simulink model "pert_test"  (R2021a)
settings: Solver=VariableStepAuto  StartTime=0.0  StopTime=10.0  RelTol=1e-3
libraries: spsDistributedParametersLineLib x23, spsThreePhaseSeriesRLCLoadLib x10, spsThreePhaseVIMeasurementLib x2, spsGroundLib x1, spsThreePhaseSourceLib x1, spsSeriesRLCBranchLib x1, spspowerguiLib x1
settings Model: Creator=Admin  LastModifiedBy=Admin

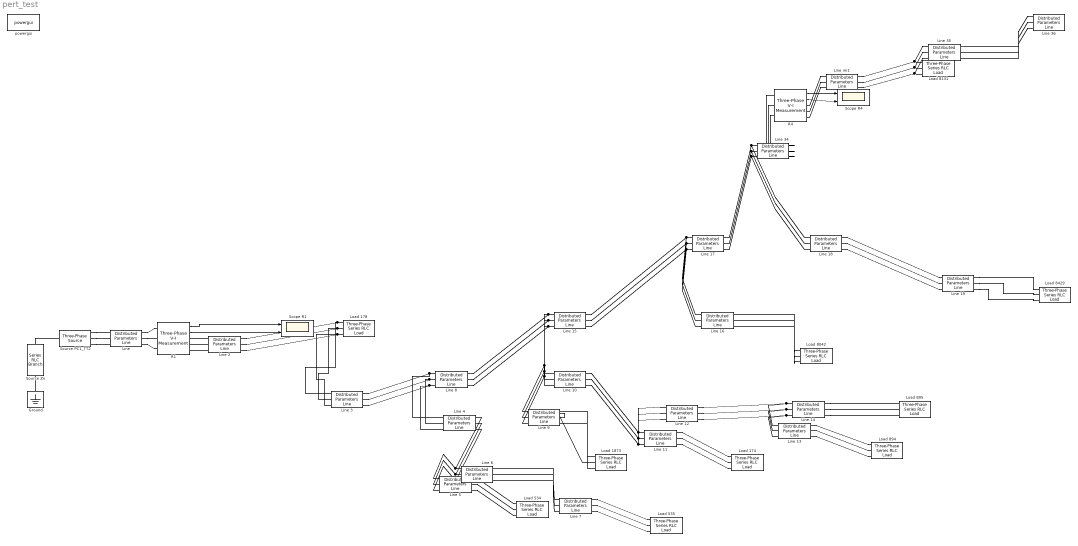
== system pert_test ==
  Ground : spsGroundLib/Ground  LConnTagsString=a
  Line : spsDistributedParametersLineLib/Distributed Parameters Line  Phases=3  Length=0.01  Frequency=50  Resistance=[0.476003738225748 0.351747138225748 0.351747138225748;0.351747138225748 0.476003738225748 0.351747138225748;0.351747138225748 0.351747138225748 0.476003738225748]  Inductance=[0.000705954362986426 0.000459934243504405 0.000459934243504405;0.000459934243504405 0.000705954362986426 0.000459934243504405;0.000459934243504405 0.000459934243504405 0.000705954362986426]  Capacitance=[5.7561313269996e-07 -1.37543883484145e-07 -1.37543912800485e-07;-1.37543883484145e-07 5.75613027339387e-07 -1.37543875208088e-07;-1.37543912800485e-07 -1.37543875208088e-07 5.75613005057695e-07]  x1=[0.0411142303390509 8948.31210962418 8947.00376137828;314.159265358979 314.159265358979 314.159265358979;0.611923927431942 -0.18676884033554 -1.75807236900485]  x2=[0.0414032445747134 8946.36312269012 8945.04836899278;314.159265358979 314.159265358979 314.159265358979;0.601696966026441 -0.186737497564286 -1.75804144074362]  x3=[0.0398944700946316 1024.91732359745 1027.78972143796;314.159265358979 314.159265358979 314.159265358979;-0.758331171111026 1.94809969608719 0.380951756978552]  x4=[0.0396805412633415 1741.95820546104 1746.36504307517;314.159265358979 314.159265358979 314.159265358979;2.35558471923768 -0.707167616201734 -2.27711571538718]  x5=2.2104317621921e-07  V1=[9.635 6853 6854;314.2 314.2 314.2;-1.242 -0.5939 -2.165]  V2=[9.699 6846 6847;314.2 314.2 314.2;-1.252 -0.5942 -2.166]  I1=[9.527 4746 4750;314.2 314.2 314.2;-2.657 2.284 0.7135]  I2=[9.488 5462 5466;314.2 314.2 314.2;0.457 -0.8227 -2.393]  nHarmo=1  Measurements=None  Decoupling=off  VsMag0=0  VrMag0=0  VsAngle0=0  VrAngle0=0  IsMag0=0  IrMag0=0  IsAngle0=0  IrAngle0=0
      settings: SourceProductBaseCode=PS
  Line 10 : spsDistributedParametersLineLib/Distributed Parameters Line  Phases=3  Length=0.16001  Frequency=50  Resistance=[0.646656091154803 0.0486237908083191 0.0486712220507153;0.0486237908083191 0.646561225344642 0.0486237934466192;0.0486712220507153 0.0486237934466192 0.646656091154803]  Inductance=[0.00282448912315926 0.00133270803418135 0.00132951476746136;0.00133270803418135 0.00282479813276775 0.00133799988507366;0.00132951476746136 0.00133799988507366 0.00282448912315926]  Capacitance=[7.89543174552926e-09 -1.85986777702161e-09 -1.7901190036642e-09;-1.85986777702161e-09 7.82540023894543e-09 -1.8957321828871e-09;-1.7901190036642e-09 -1.8957321828871e-09 7.91264394645417e-09]  x1=[149.213225790778 5073.09179697526 5075.1684030107;314.159265358979 314.159265358979 314.159265358979;0.854381593501133 -0.358879184977843 -1.9302938601983]  x2=[149.213871626029 5073.02522515298 5075.10194812837;314.159265358979 314.159265358979 314.159265358979;0.854382399962997 -0.358882672030428 -1.93029730927887]  x3=[0.131685687254381 12.3901652064539 12.4941973747481;314.159265358979 314.159265358979 314.159265358979;0.840457441539283 -0.340918292447417 -1.91251905202151]  x4=[0.129244563248061 13.4297587319227 13.5345752277212;314.159265358979 314.159265358979 314.159265358979;0.868326429129559 -0.375636900721885 -1.94688971846806]  x5=7.6668354874491e-07  V1=[104 5068 5071;314.2 314.2 314.2;0.347 -0.922 -2.492]  V2=[104 5068 5071;314.2 314.2 314.2;0.347 -0.922 -2.492]  I1=[0.09471 11.28 11.38;314.2 314.2 314.2;0.3017 -0.8557 -2.427]  I2=[0.0873 14.56 14.67;314.2 314.2 314.2;0.3959 -0.9736 -2.543]  nHarmo=1  Measurements=None  Decoupling=off  VsMag0=0  VrMag0=0  VsAngle0=0  VrAngle0=0  IsMag0=0  IrMag0=0  IsAngle0=0  IrAngle0=0
      settings: SourceProductBaseCode=PS
  Line 11 : spsDistributedParametersLineLib/Distributed Parameters Line  Phases=3  Length=0.16  Frequency=50  Resistance=[0.646656091154803 0.0486237908083191 0.0486712220507153;0.0486237908083191 0.646561225344642 0.0486237934466192;0.0486712220507153 0.0486237934466192 0.646656091154803]  Inductance=[0.00282448912315926 0.00133270803418135 0.00132951476746136;0.00133270803418135 0.00282479813276775 0.00133799988507366;0.00132951476746136 0.00133799988507366 0.00282448912315926]  Capacitance=[7.89543174552926e-09 -1.85986777702161e-09 -1.7901190036642e-09;-1.85986777702161e-09 7.82540023894543e-09 -1.8957321828871e-09;-1.7901190036642e-09 -1.8957321828871e-09 7.91264394645417e-09]  x1=[149.213871626029 5073.02522515298 5075.10194812837;314.159265358979 314.159265358979 314.159265358979;0.854382415015852 -0.358882660071923 -1.93029729730898]  x2=[149.214171090953 5072.98211898509 5075.05891133273;314.159265358979 314.159265358979 314.159265358979;0.854383159423688 -0.358884111107554 -1.93029872085362]  x3=[0.131190371118207 12.5931840643473 12.6973813420866;314.159265358979 314.159265358979 314.159265358979;0.84839334316163 -0.345374078320807 -1.91690149404068]  x4=[0.12971992179425 13.2248523824609 13.3295300528108;314.159265358979 314.159265358979 314.159265358979;0.860197908716152 -0.371934178623254 -1.94324615089134]  x5=7.66635634017784e-07  V1=[104 5068 5071;314.2 314.2 314.2;0.347 -0.922 -2.492]  V2=[104 5068 5071;314.2 314.2 314.2;0.347 -0.922 -2.492]  I1=[0.09332 11.85 11.95;314.2 314.2 314.2;0.3203 -0.879 -2.45]  I2=[0.08855 13.96 14.07;314.2 314.2 314.2;0.375 -0.9588 -2.529]  nHarmo=1  Measurements=None  Decoupling=off  VsMag0=0  VrMag0=0  VsAngle0=0  VrAngle0=0  IsMag0=0  IrMag0=0  IsAngle0=0  IrAngle0=0
      settings: SourceProductBaseCode=PS
  Line 12 : spsDistributedParametersLineLib/Distributed Parameters Line  Phases=3  Length=0.18  Frequency=50  Resistance=[0.646656091154803 0.0486237908083191 0.0486712220507153;0.0486237908083191 0.646561225344642 0.0486237934466192;0.0486712220507153 0.0486237934466192 0.646656091154803]  Inductance=[0.00282448912315926 0.00133270803418135 0.00132951476746136;0.00133270803418135 0.00282479813276775 0.00133799988507366;0.00132951476746136 0.00133799988507366 0.00282448912315926]  Capacitance=[7.89543174552926e-09 -1.85986777702161e-09 -1.7901190036642e-09;-1.85986777702161e-09 7.82540023894543e-09 -1.8957321828871e-09;-1.7901190036642e-09 -1.8957321828871e-09 7.91264394645417e-09]  x1=[149.213871626029 5073.02522515298 5075.10194812837;314.159265358979 314.159265358979 314.159265358979;0.854352309304904 -0.358906577081988 -1.93032123708634]  x2=[149.214246032471 5072.99850455641 5075.07528028043;314.159265358979 314.159265358979 314.159265358979;0.854352423026501 -0.358908785554651 -1.9303234330767]  x3=[0.130940881276861 12.7037241385656 12.808012867364;314.159265358979 314.159265358979 314.159265358979;0.846589788692399 -0.354586333911735 -1.92606814160609]  x4=[0.1299700382589 13.1117349542385 13.216325469339;314.159265358979 314.159265358979 314.159265358979;0.861900957888328 -0.363306474700014 -1.93465724067612]  x5=8.62465088270006e-07  V1=[104 5068 5071;314.2 314.2 314.2;0.347 -0.9221 -2.492]  V2=[104 5068 5071;314.2 314.2 314.2;0.347 -0.9221 -2.492]  I1=[0.09224 12.31 12.42;314.2 314.2 314.2;0.3278 -0.9025 -2.473]  I2=[0.08959 13.48 13.59;314.2 314.2 314.2;0.3665 -0.9401 -2.51]  nHarmo=1  Measurements=None  Decoupling=off  VsMag0=0  VrMag0=0  VsAngle0=0  VrAngle0=0  IsMag0=0  IrMag0=0  IsAngle0=0  IrAngle0=0
      settings: SourceProductBaseCode=PS
  Line 13 : spsDistributedParametersLineLib/Distributed Parameters Line  Phases=3  Length=0.52999  Frequency=50  Resistance=[0.646656091154803 0.0486237908083191 0.0486712220507153;0.0486237908083191 0.646561225344642 0.0486237934466192;0.0486712220507153 0.0486237934466192 0.646656091154803]  Inductance=[0.00282448912315926 0.00133270803418135 0.00132951476746136;0.00133270803418135 0.00282479813276775 0.00133799988507366;0.00132951476746136 0.00133799988507366 0.00282448912315926]  Capacitance=[7.89543174552926e-09 -1.85986777702161e-09 -1.7901190036642e-09;-1.85986777702161e-09 7.82540023894543e-09 -1.8957321828871e-09;-1.7901190036642e-09 -1.8957321828871e-09 7.91264394645417e-09]  x1=[149.214246032471 5072.99850455641 5075.07528028043;314.159265358979 314.159265358979 314.159265358979;0.853825588137772 -0.359327321272278 -1.93074236721069]  x2=[149.214759137192 5072.93165456291 5075.00854514023;314.159265358979 314.159265358979 314.159265358979;0.853826575807285 -0.35932955267529 -1.93074455793964]  x3=[0.130771017383896 12.7549372431025 12.859183235875;314.159265358979 314.159265358979 314.159265358979;0.850251507542855 -0.353345601060044 -1.92481481091205]  x4=[0.130089920102991 13.0502325975811 13.1547040549009;314.159265358979 314.159265358979 314.159265358979;0.856619427944257 -0.365802638446214 -1.93716631883698]  x5=2.53943262295678e-06  V1=[104 5068 5071;314.2 314.2 314.2;0.3465 -0.9225 -2.493]  V2=[104 5068 5071;314.2 314.2 314.2;0.3465 -0.9225 -2.493]  I1=[0.09195 12.42 12.53;314.2 314.2 314.2;0.3337 -0.9048 -2.475]  I2=[0.08984 13.36 13.47;314.2 314.2 314.2;0.3587 -0.9395 -2.51]  nHarmo=1  Measurements=None  Decoupling=off  VsMag0=0  VrMag0=0  VsAngle0=0  VrAngle0=0  IsMag0=0  IrMag0=0  IsAngle0=0  IrAngle0=0
      settings: SourceProductBaseCode=PS
  Line 14 : spsDistributedParametersLineLib/Distributed Parameters Line  Phases=3  Length=2.16  Frequency=50  Resistance=[0.646656091154803 0.0486237908083191 0.0486712220507153;0.0486237908083191 0.646561225344642 0.0486237934466192;0.0486712220507153 0.0486237934466192 0.646656091154803]  Inductance=[0.00282448912315926 0.00133270803418135 0.00132951476746136;0.00133270803418135 0.00282479813276775 0.00133799988507366;0.00132951476746136 0.00133799988507366 0.00282448912315926]  Capacitance=[7.89543174552926e-09 -1.85986777702161e-09 -1.7901190036642e-09;-1.85986777702161e-09 7.82540023894543e-09 -1.8957321828871e-09;-1.7901190036642e-09 -1.8957321828871e-09 7.91264394645417e-09]  x1=[149.214246032471 5072.99850455641 5075.07528028043;314.159265358979 314.159265358979 314.159265358979;0.851371957642685 -0.361276569551057 -1.93269347103581]  x2=[149.215599745592 5072.92782202238 5075.00471058088;314.159265358979 314.159265358979 314.159265358979;0.851372325805624 -0.361288337822401 -1.93270520756816]  x3=[0.130471845940392 12.8222586614419 12.9262085967551;314.159265358979 314.159265358979 314.159265358979;0.847437720908756 -0.36272928606629 -1.93415855249805]  x4=[0.130182602840782 12.9344765550706 13.0384987184158;314.159265358979 314.159265358979 314.159265358979;0.852059134294189 -0.36242211883212 -1.93382918659383]  x5=1.03495810592401e-05  V1=[104 5068 5071;314.2 314.2 314.2;0.344 -0.9244 -2.495]  V2=[104 5068 5071;314.2 314.2 314.2;0.344 -0.9245 -2.495]  I1=[0.09108 12.75 12.85;314.2 314.2 314.2;0.3377 -0.9226 -2.493]  I2=[0.09055 12.98 13.09;314.2 314.2 314.2;0.347 -0.9288 -2.499]  nHarmo=1  Measurements=None  Decoupling=off  VsMag0=0  VrMag0=0  VsAngle0=0  VrAngle0=0  IsMag0=0  IrMag0=0  IsAngle0=0  IrAngle0=0
      settings: SourceProductBaseCode=PS
  Line 15 : spsDistributedParametersLineLib/Distributed Parameters Line  Phases=3  Length=4.0599  Frequency=50  Resistance=[0.502970710632245 0.0486237908083191 0.0486712220507153;0.0486237908083191 0.502875844822084 0.0486237934466192;0.0486712220507153 0.0486237934466192 0.502970710632245]  Inductance=[0.00286900545038753 0.00133270803418135 0.00132951476746136;0.00133270803418135 0.00286931445999602 0.00133799988507366;0.00132951476746136 0.00133799988507366 0.00286900545038753]  Capacitance=[8.11484299003193e-09 -1.94249816214699e-09 -1.86930692621136e-09;-1.94249816214699e-09 8.0425699231653e-09 -1.98049571960044e-09;-1.86930692621136e-09 -1.98049571960044e-09 8.13337738722527e-09]  x1=[202.750210342539 5073.03837892235 5074.76675240275;314.159265358979 314.159265358979 314.159265358979;0.83429930014509 -0.357482686995033 -1.92888716041959]  x2=[196.119997886971 1701.47554123724 1705.23871567303;314.159265358979 314.159265358979 314.159265358979;0.764111011186659 -0.810138203895518 -2.37983068117659]  x3=[1.90070350685825 1329.93326863877 1333.43957927887;314.159265358979 314.159265358979 314.159265358979;-2.4653689123904 2.16858567634875 0.600235252254855]  x4=[2.24763170484556 1344.74738403574 1348.40388504844;314.159265358979 314.159265358979 314.159265358979;0.694889905792329 -0.96698721867378 -2.53533333902708]  x5=1.96600110340104e-05  V1=[157.3 5068 5071;314.2 314.2 314.2;0.3043 -0.9206 -2.491]  V2=[157.3 5040 5043;314.2 314.2 314.2;0.3032 -0.924 -2.494]  I1=[0.117 3.332 3.375;314.2 314.2 314.2;0.2152 0.2769 -1.319]  I2=[0.1593 24.64 24.76;314.2 314.2 314.2;0.3633 -1.051 -2.621]  nHarmo=1  Measurements=None  Decoupling=off  VsMag0=0  VrMag0=0  VsAngle0=0  VrAngle0=0  IsMag0=0  IrMag0=0  IsAngle0=0  IrAngle0=0
      settings: SourceProductBaseCode=PS
  Line 16 : spsDistributedParametersLineLib/Distributed Parameters Line  Phases=3  Length=0.01  Frequency=50  Resistance=[0.646656091154803 0.0486237908083191 0.0486712220507153;0.0486237908083191 0.646561225344642 0.0486237934466192;0.0486712220507153 0.0486237934466192 0.646656091154803]  Inductance=[0.00282448912315926 0.00133270803418135 0.00132951476746136;0.00133270803418135 0.00282479813276775 0.00133799988507366;0.00132951476746136 0.00133799988507366 0.00282448912315926]  Capacitance=[7.89543174552926e-09 -1.85986777702161e-09 -1.7901190036642e-09;-1.85986777702161e-09 7.82540023894543e-09 -1.8957321828871e-09;-1.7901190036642e-09 -1.8957321828871e-09 7.91264394645417e-09]  x1=[179.885070085177 1701.46709294524 1705.86748938584;314.159265358979 314.159265358979 314.159265358979;0.811091080789274 -0.811236684304932 -2.38098616023635]  x2=[179.885070941273 1701.46697906805 1705.86737546575;314.159265358979 314.159265358979 314.159265358979;0.811091080606212 -0.811236696501084 -2.38098617221768]  x3=[0.157295515004497 4.31654315587841 4.36104659562899;314.159265358979 314.159265358979 314.159265358979;0.810812578153983 -0.809595891011948 -2.37935939465627]  x4=[0.157262577718036 4.34346334451761 4.38804158294889;314.159265358979 314.159265358979 314.159265358979;0.811354587209658 -0.812879241827761 -2.38261486309864]  x5=4.79147271261115e-08  V1=[104.3 5040 5044;314.2 314.2 314.2;0.347 -0.9253 -2.495]  V2=[104.3 5040 5044;314.2 314.2 314.2;0.347 -0.9253 -2.495]  I1=[0.09135 12.75 12.86;314.2 314.2 314.2;0.3451 -0.9225 -2.493]  I2=[0.09103 12.9 13.01;314.2 314.2 314.2;0.3489 -0.928 -2.498]  nHarmo=1  Measurements=None  Decoupling=off  VsMag0=0  VrMag0=0  VsAngle0=0  VrAngle0=0  IsMag0=0  IrMag0=0  IsAngle0=0  IrAngle0=0
      settings: SourceProductBaseCode=PS
  Line 17 : spsDistributedParametersLineLib/Distributed Parameters Line  Phases=3  Length=0.35001  Frequency=50  Resistance=[0.646656091154803 0.0486237908083191 0.0486712220507153;0.0486237908083191 0.646561225344642 0.0486237934466192;0.0486712220507153 0.0486237934466192 0.646656091154803]  Inductance=[0.00282448912315926 0.00133270803418135 0.00132951476746136;0.00133270803418135 0.00282479813276775 0.00133799988507366;0.00132951476746136 0.00133799988507366 0.00282448912315926]  Capacitance=[7.89543174552926e-09 -1.85986777702161e-09 -1.7901190036642e-09;-1.85986777702161e-09 7.82540023894543e-09 -1.8957321828871e-09;-1.7901190036642e-09 -1.8957321828871e-09 7.91264394645417e-09]  x1=[179.885070085177 1701.46709294524 1705.86748938584;314.159265358979 314.159265358979 314.159265358979;0.810579268650308 -0.811643285434538 -2.38139314842144]  x2=[182.371745576672 1400.00068456796 1403.96945961588;314.159265358979 314.159265358979 314.159265358979;0.814731037765984 -0.936371518002843 -2.5053725610288]  x3=[4.06178609523338 1339.01105266299 1342.62523270451;314.159265358979 314.159265358979 314.159265358979;-0.0277823504523922 2.17198710182874 0.603610171359378]  x4=[3.85767553746922 1346.84534468075 1350.54199114166;314.159265358979 314.159265358979 314.159265358979;3.05263358310844 -0.969013375221598 -2.53739188572418]  x5=1.67706336414103e-06  V1=[104.3 5040 5044;314.2 314.2 314.2;0.3465 -0.9257 -2.496]  V2=[104.3 5037 5041;314.2 314.2 314.2;0.3465 -0.9259 -2.496]  I1=[0.1199 3.328 3.373;314.2 314.2 314.2;0.1188 0.2711 -1.325]  I2=[0.0709 24.62 24.74;314.2 314.2 314.2;0.7375 -1.052 -2.622]  nHarmo=1  Measurements=None  Decoupling=off  VsMag0=0  VrMag0=0  VsAngle0=0  VrAngle0=0  IsMag0=0  IrMag0=0  IsAngle0=0  IrAngle0=0
      settings: SourceProductBaseCode=PS
  Line 18 : spsDistributedParametersLineLib/Distributed Parameters Line  Phases=3  Length=0.26  Frequency=50  Resistance=[0.646656091154803 0.0486237908083191 0.0486712220507153;0.0486237908083191 0.646561225344642 0.0486237934466192;0.0486712220507153 0.0486237934466192 0.646656091154803]  Inductance=[0.00282448912315926 0.00133270803418135 0.00132951476746136;0.00133270803418135 0.00282479813276775 0.00133799988507366;0.00132951476746136 0.00133799988507366 0.00282448912315926]  Capacitance=[7.89543174552926e-09 -1.85986777702161e-09 -1.7901190036642e-09;-1.85986777702161e-09 7.82540023894543e-09 -1.8957321828871e-09;-1.7901190036642e-09 -1.8957321828871e-09 7.91264394645417e-09]  x1=[182.371745576672 1400.00068456796 1403.96945961588;314.159265358979 314.159265358979 314.159265358979;0.814866528518104 -0.936263879499047 -2.50526482006077]  x2=[182.388454420939 1399.94621323615 1403.91462108741;314.159265358979 314.159265358979 314.159265358979;0.814838051461898 -0.936358387460504 -2.50535894780343]  x3=[0.167086189047892 2.95333256988402 2.98922060238648;314.159265358979 314.159265358979 314.159265358979;0.599412383613478 -1.05721683792705 -2.62515322548885]  x4=[0.159690410997041 4.20668526142641 4.24568050071062;314.159265358979 314.159265358979 314.159265358979;1.04003772145386 -0.851797804445089 -2.42130309548101]  x5=1.2457829052789e-06  V1=[104.3 5037 5041;314.2 314.2 314.2;0.3467 -0.9258 -2.496]  V2=[104.3 5037 5040;314.2 314.2 314.2;0.3467 -0.9259 -2.496]  I1=[0.1068 7.796 7.899;314.2 314.2 314.2;0.212 -0.9318 -2.502]  I2=[0.0779 17.83 17.94;314.2 314.2 314.2;0.5314 -0.9235 -2.494]  nHarmo=1  Measurements=None  Decoupling=off  VsMag0=0  VrMag0=0  VsAngle0=0  VrAngle0=0  IsMag0=0  IrMag0=0  IsAngle0=0  IrAngle0=0
      settings: SourceProductBaseCode=PS
  Line 19 : spsDistributedParametersLineLib/Distributed Parameters Line  Phases=3  Length=0.03  Frequency=50  Resistance=[0.476003738225748 0.351747138225748 0.351747138225748;0.351747138225748 0.476003738225748 0.351747138225748;0.351747138225748 0.351747138225748 0.476003738225748]  Inductance=[0.000705954362986426 0.000459934243504405 0.000459934243504405;0.000459934243504405 0.000705954362986426 0.000459934243504405;0.000459934243504405 0.000459934243504405 0.000705954362986426]  Capacitance=[5.7561313269996e-07 -1.37543883484145e-07 -1.37543912800485e-07;-1.37543883484145e-07 5.75613027339387e-07 -1.37543875208088e-07;-1.37543912800485e-07 -1.37543875208088e-07 5.75613005057695e-07]  x1=[167.303090496688 1399.94770504645 1404.02596945619;314.159265358979 314.159265358979 314.159265358979;0.872359281453115 -0.854508142548132 -2.42365911950902]  x2=[167.30361520206 1399.94617123627 1404.02443171602;314.159265358979 314.159265358979 314.159265358979;0.872351907392031 -0.854510119373181 -2.4236610974484]  x3=[2.27383652219201 74.7334923771782 74.9511143973152;314.159265358979 314.159265358979 314.159265358979;0.856968163497245 -0.859264063481118 -2.42841994721498]  x4=[2.27429011017898 75.9925043523949 76.2139622623068;314.159265358979 314.159265358979 314.159265358979;0.887531623643366 -0.849956787434816 -2.41910295030125]  x5=6.63129528657629e-07  V1=[39.29 5037 5041;314.2 314.2 314.2;0.4733 -0.844 -2.414]  V2=[39.29 5037 5041;314.2 314.2 314.2;0.4733 -0.844 -2.414]  I1=[0.5337 266.1 266.4;314.2 314.2 314.2;0.4559 -0.8442 -2.414]  I2=[0.5344 276.2 276.4;314.2 314.2 314.2;0.4906 -0.844 -2.414]  nHarmo=1  Measurements=None  Decoupling=off  VsMag0=0  VrMag0=0  VsAngle0=0  VrAngle0=0  IsMag0=0  IrMag0=0  IsAngle0=0  IrAngle0=0
      settings: SourceProductBaseCode=PS
  Line 2 : spsDistributedParametersLineLib/Distributed Parameters Line  Phases=3  Length=0.61194  Frequency=50  Resistance=[0.502970710632245 0.0486237908083191 0.0486712220507153;0.0486237908083191 0.502875844822084 0.0486237934466192;0.0486712220507153 0.0486237934466192 0.502970710632245]  Inductance=[0.00286900545038753 0.00133270803418135 0.00132951476746136;0.00133270803418135 0.00286931445999602 0.00133799988507366;0.00132951476746136 0.00133799988507366 0.00286900545038753]  Capacitance=[8.11484299003193e-09 -1.94249816214699e-09 -1.86930692621136e-09;-1.94249816214699e-09 8.0425699231653e-09 -1.98049571960044e-09;-1.86930692621136e-09 -1.98049571960044e-09 8.13337738722527e-09]  x1=[210.953435908036 8945.04573307882 8943.50461999697;314.159265358979 314.159265358979 314.159265358979;0.910242629519443 -0.262856842111434 -1.83436216672367]  x2=[209.749296194644 8402.41986133134 8401.34045297359;314.159265358979 314.159265358979 314.159265358979;0.900717553251165 -0.270465431561692 -1.8419653678465]  x3=[1.90102560594307 1328.15456729144 1331.62038060609;314.159265358979 314.159265358979 314.159265358979;-2.46541318627011 2.16790069865186 0.599542816366069]  x4=[2.26185132853584 1362.02834016226 1365.83906812946;314.159265358979 314.159265358979 314.159265358979;0.713186877842024 -0.95264219249401 -2.52097875708587]  x5=2.96331120277651e-06  V1=[159.9 6845 6846;314.2 314.2 314.2;0.4431 -0.6704 -2.242]  V2=[157.3 5087 5090;314.2 314.2 314.2;0.3101 -0.9143 -2.485]  I1=[17.14 5085 5089;314.2 314.2 314.2;-2.556 2.225 0.6553]  I2=[17.41 5115 5119;314.2 314.2 314.2;0.5825 -0.9156 -2.485]  nHarmo=1  Measurements=None  Decoupling=off  VsMag0=0  VrMag0=0  VsAngle0=0  VrAngle0=0  IsMag0=0  IrMag0=0  IsAngle0=0  IrAngle0=0
      settings: SourceProductBaseCode=PS
  Line 3 : spsDistributedParametersLineLib/Distributed Parameters Line  Phases=3  Length=2.5878  Frequency=50  Resistance=[0.502970710632245 0.0486237908083191 0.0486712220507153;0.0486237908083191 0.502875844822084 0.0486237934466192;0.0486712220507153 0.0486237934466192 0.502970710632245]  Inductance=[0.00286900545038753 0.00133270803418135 0.00132951476746136;0.00133270803418135 0.00286931445999602 0.00133799988507366;0.00132951476746136 0.00133799988507366 0.00286900545038753]  Capacitance=[8.11484299003193e-09 -1.94249816214699e-09 -1.86930692621136e-09;-1.94249816214699e-09 8.0425699231653e-09 -1.98049571960044e-09;-1.86930692621136e-09 -1.98049571960044e-09 8.13337738722527e-09]  x1=[209.749296194644 8402.41986133134 8401.3404529736;314.159265358979 314.159265358979 314.159265358979;0.897711653706009 -0.272899822966975 -1.84440249888836]  x2=[204.872544447172 6115.88361830447 6116.74102091159;314.159265358979 314.159265358979 314.159265358979;0.856234287812334 -0.319959251953308 -1.89141397681942]  x3=[1.90045537890804 1327.40499524336 1330.86530567937;314.159265358979 314.159265358979 314.159265358979;-2.46748381849127 2.16622429551194 0.597865063932338]  x4=[2.25750610846255 1356.25171972731 1360.0052772911;314.159265358979 314.159265358979 314.159265358979;0.706257545934117 -0.95824951925633 -2.52659181932282]  x5=1.25313866237622e-05  V1=[157.3 5087 5090;314.2 314.2 314.2;0.3098 -0.9146 -2.485]  V2=[157.3 5078 5081;314.2 314.2 314.2;0.3094 -0.9156 -2.486]  I1=[0.1093 6.229 6.183;314.2 314.2 314.2;0.1996 1.242 -0.3409]  I2=[0.1676 29.77 29.89;314.2 314.2 314.2;0.3802 -1.091 -2.661]  nHarmo=1  Measurements=None  Decoupling=off  VsMag0=0  VrMag0=0  VsAngle0=0  VrAngle0=0  IsMag0=0  IrMag0=0  IsAngle0=0  IrAngle0=0
      settings: SourceProductBaseCode=PS
  Line 34 : spsDistributedParametersLineLib/Distributed Parameters Line  Phases=3  Length=0.35001  Frequency=50  Resistance=[0.646656091154803 0.0486237908083191 0.0486712220507153;0.0486237908083191 0.646561225344642 0.0486237934466192;0.0486712220507153 0.0486237934466192 0.646656091154803]  Inductance=[0.00282448912315926 0.00133270803418135 0.00132951476746136;0.00133270803418135 0.00282479813276775 0.00133799988507366;0.00132951476746136 0.00133799988507366 0.00282448912315926]  Capacitance=[7.89543174552926e-09 -1.85986777702161e-09 -1.7901190036642e-09;-1.85986777702161e-09 7.82540023894543e-09 -1.8957321828871e-09;-1.7901190036642e-09 -1.8957321828871e-09 7.91264394645417e-09]  x1=[182.371745576672 1400.00068456796 1403.96945961588;314.159265358979 314.159265358979 314.159265358979;0.815149857879689 -0.936038792929776 -2.50503951922502]  x2=[182.877451789185 1341.60539243015 1345.4535146162;314.159265358979 314.159265358979 314.159265358979;0.81599519711756 -0.968372178453613 -2.53717061637905]  x3=[4.03393861950928 1339.3914946764 1343.0141833016;314.159265358979 314.159265358979 314.159265358979;-0.0216449431923269 2.17245710038757 0.604081023647271]  x4=[3.82747454993201 1346.36606825415 1350.06243406906;314.159265358979 314.159265358979 314.159265358979;3.05793810228926 -0.969046280054018 -2.53742440744983]  x5=3.4391753689309e-07  V1=[104.3 5037 5041;314.2 314.2 314.2;0.3465 -0.9259 -2.496]  V2=[104.3 5036 5039;314.2 314.2 314.2;0.3466 -0.926 -2.496]  I1=[0.103 6.978 7.072;314.2 314.2 314.2;0.2231 -0.4579 -2.033]  I2=[0.08118 19.65 19.77;314.2 314.2 314.2;0.5028 -1.087 -2.657]  nHarmo=1  Measurements=None  Decoupling=off  VsMag0=0  VrMag0=0  VsAngle0=0  VrAngle0=0  IsMag0=0  IrMag0=0  IsAngle0=0  IrAngle0=0
      settings: SourceProductBaseCode=PS
  Line 35 : spsDistributedParametersLineLib/Distributed Parameters Line  Phases=3  Length=0.09  Frequency=50  Resistance=[0.646656091154803 0.0486237908083191 0.0486712220507153;0.0486237908083191 0.646561225344642 0.0486237934466192;0.0486712220507153 0.0486237934466192 0.646656091154803]  Inductance=[0.00282448912315926 0.00133270803418135 0.00132951476746136;0.00133270803418135 0.00282479813276775 0.00133799988507366;0.00132951476746136 0.00133799988507366 0.00282448912315926]  Capacitance=[7.89543174552926e-09 -1.85986777702161e-09 -1.7901190036642e-09;-1.85986777702161e-09 7.82540023894543e-09 -1.8957321828871e-09;-1.7901190036642e-09 -1.8957321828871e-09 7.91264394645417e-09]  x1=[182.880070226776 1341.37624017114 1345.22434166028;314.159265358979 314.159265358979 314.159265358979;0.815974718254692 -0.968443934677024 -2.53724129720897]  x2=[182.880114952442 1341.33098656065 1345.1789735001;314.159265358979 314.159265358979 314.159265358979;0.815975322808244 -0.968458238709031 -2.53725530809804]  x3=[0.160598019640175 2.72672634763799 2.76224513737563;314.159265358979 314.159265358979 314.159265358979;0.816007361414457 -0.899443355647667 -2.46795084830243]  x4=[0.159184887852889 4.11057674740326 4.14746861546078;314.159265358979 314.159265358979 314.159265358979;0.815806313555697 -1.0142960559986 -2.58347005077264]  x5=4.31232544135003e-07  V1=[104.3 5036 5039;314.2 314.2 314.2;0.347 -0.9257 -2.496]  V2=[104.3 5035 5039;314.2 314.2 314.2;0.347 -0.9257 -2.496]  I1=[0.0997 8.795 8.897;314.2 314.2 314.2;0.2278 -0.6939 -2.265]  I2=[0.08427 17.19 17.3;314.2 314.2 314.2;0.488 -1.044 -2.614]  nHarmo=1  Measurements=None  Decoupling=off  VsMag0=0  VrMag0=0  VsAngle0=0  VrAngle0=0  IsMag0=0  IrMag0=0  IsAngle0=0  IrAngle0=0
      settings: SourceProductBaseCode=PS
  Line 36 : spsDistributedParametersLineLib/Distributed Parameters Line  Phases=3  Length=0.32  Frequency=50  Resistance=[0.502970710632245 0.0486237908083191 0.0486712220507153;0.0486237908083191 0.502875844822084 0.0486237934466192;0.0486712220507153 0.0486237934466192 0.502970710632245]  Inductance=[0.00286900545038753 0.00133270803418135 0.00132951476746136;0.00133270803418135 0.00286931445999602 0.00133799988507366;0.00132951476746136 0.00133799988507366 0.00286900545038753]  Capacitance=[8.11484299003193e-09 -1.94249816214699e-09 -1.86930692621136e-09;-1.94249816214699e-09 8.0425699231653e-09 -1.98049571960044e-09;-1.86930692621136e-09 -1.98049571960044e-09 8.13337738722527e-09]  x1=[194.530873773176 1341.38256448759 1344.54741165392;314.159265358979 314.159265358979 314.159265358979;0.773103462588214 -0.962701567077333 -2.53148168759744]  x2=[194.529311157478 1341.25256635573 1344.4170348619;314.159265358979 314.159265358979 314.159265358979;0.773102073828493 -0.962761112616204 -2.53154030662713]  x3=[0.16930943018757 2.72800917025858 2.76184155276116;314.159265358979 314.159265358979 314.159265358979;0.786828015750819 -0.893646383545178 -2.46211290866461]  x4=[0.171915330341933 4.11159048747675 4.14671311001747;314.159265358979 314.159265358979 314.159265358979;0.759102431514948 -1.00887603858421 -2.57804029905519]  x5=1.54959568730346e-06  V1=[157.3 5035 5038;314.2 314.2 314.2;0.3089 -0.9198 -2.49]  V2=[157.3 5034 5037;314.2 314.2 314.2;0.3088 -0.9198 -2.49]  I1=[0.1289 8.799 8.901;314.2 314.2 314.2;0.2954 -0.688 -2.259]  I2=[0.147 17.19 17.3;314.2 314.2 314.2;0.3202 -1.038 -2.608]  nHarmo=1  Measurements=None  Decoupling=off  VsMag0=0  VrMag0=0  VsAngle0=0  VrAngle0=0  IsMag0=0  IrMag0=0  IsAngle0=0  IrAngle0=0
      settings: SourceProductBaseCode=PS
  Line 4 : spsDistributedParametersLineLib/Distributed Parameters Line  Phases=3  Length=0.53  Frequency=50  Resistance=[0.502970710632245 0.0486237908083191 0.0486712220507153;0.0486237908083191 0.502875844822084 0.0486237934466192;0.0486712220507153 0.0486237934466192 0.502970710632245]  Inductance=[0.00286900545038753 0.00133270803418135 0.00132951476746136;0.00133270803418135 0.00286931445999602 0.00133799988507366;0.00132951476746136 0.00133799988507366 0.00286900545038753]  Capacitance=[8.11484299003193e-09 -1.94249816214699e-09 -1.86930692621136e-09;-1.94249816214699e-09 8.0425699231653e-09 -1.98049571960044e-09;-1.86930692621136e-09 -1.98049571960044e-09 8.13337738722527e-09]  x1=[204.872544447172 6115.88361830447 6116.74102091159;314.159265358979 314.159265358979 314.159265358979;0.859364843663468 -0.31742390499867 -1.88887577661397]  x2=[204.872907593175 6115.37930863852 6116.23759521471;314.159265358979 314.159265358979 314.159265358979;0.859351660366052 -0.317469186750529 -1.88892068013246]  x3=[0.17715314379777 14.0194534986931 14.1404423348181;314.159265358979 314.159265358979 314.159265358979;0.851848941706149 -0.281655607996968 -1.85345256647412]  x4=[0.182158196604418 17.1264931095556 17.2488773726934;314.159265358979 314.159265358979 314.159265358979;0.865865956636945 -0.347336124727681 -1.91854906094429]  x5=2.56651785709636e-06  V1=[157.3 5078 5081;314.2 314.2 314.2;0.31 -0.9152 -2.485]  V2=[157.3 5077 5080;314.2 314.2 314.2;0.31 -0.9152 -2.486]  I1=[0.1333 10.2 10.3;314.2 314.2 314.2;0.305 -0.7979 -2.369]  I2=[0.1426 15.76 15.87;314.2 314.2 314.2;0.3139 -0.9915 -2.561]  nHarmo=1  Measurements=None  Decoupling=off  VsMag0=0  VrMag0=0  VsAngle0=0  VrAngle0=0  IsMag0=0  IrMag0=0  IsAngle0=0  IrAngle0=0
      settings: SourceProductBaseCode=PS
  Line 5 : spsDistributedParametersLineLib/Distributed Parameters Line  Phases=3  Length=0.26  Frequency=50  Resistance=[0.502970710632245 0.0486237908083191 0.0486712220507153;0.0486237908083191 0.502875844822084 0.0486237934466192;0.0486712220507153 0.0486237934466192 0.502970710632245]  Inductance=[0.00286900545038753 0.00133270803418135 0.00132951476746136;0.00133270803418135 0.00286931445999602 0.00133799988507366;0.00132951476746136 0.00133799988507366 0.00286900545038753]  Capacitance=[8.11484299003193e-09 -1.94249816214699e-09 -1.86930692621136e-09;-1.94249816214699e-09 8.0425699231653e-09 -1.98049571960044e-09;-1.86930692621136e-09 -1.98049571960044e-09 8.13337738722527e-09]  x1=[204.872907593175 6115.37930863852 6116.23759521471;314.159265358979 314.159265358979 314.159265358979;0.859762414608351 -0.31713652872849 -1.88858764774084]  x2=[204.872684284688 6115.2117855552 6116.07043301869;314.159265358979 314.159265358979 314.159265358979;0.859758814239138 -0.317147297751536 -1.88859830495027]  x3=[0.178056481137305 14.6318188611666 14.7531006651495;314.159265358979 314.159265358979 314.159265358979;0.859214228136178 -0.286779673970788 -1.85849753635592]  x4=[0.181284371993384 16.5159329833022 16.6381770498057;314.159265358979 314.159265358979 314.159265358979;0.859905238895954 -0.344341656037937 -1.91558033377114]  x5=1.25904649593406e-06  V1=[157.3 5077 5080;314.2 314.2 314.2;0.3104 -0.9149 -2.485]  V2=[157.3 5076 5079;314.2 314.2 314.2;0.3104 -0.9149 -2.485]  I1=[0.1348 11.11 11.21;314.2 314.2 314.2;0.3109 -0.8343 -2.405]  I2=[0.1411 14.8 14.91;314.2 314.2 314.2;0.3096 -0.9756 -2.545]  nHarmo=1  Measurements=None  Decoupling=off  VsMag0=0  VrMag0=0  VsAngle0=0  VrAngle0=0  IsMag0=0  IrMag0=0  IsAngle0=0  IrAngle0=0
      settings: SourceProductBaseCode=PS
  Line 6 : spsDistributedParametersLineLib/Distributed Parameters Line  Phases=3  Length=0.06  Frequency=50  Resistance=[0.502970710632245 0.0486237908083191 0.0486712220507153;0.0486237908083191 0.502875844822084 0.0486237934466192;0.0486712220507153 0.0486237934466192 0.502970710632245]  Inductance=[0.00286900545038753 0.00133270803418135 0.00132951476746136;0.00133270803418135 0.00286931445999602 0.00133799988507366;0.00132951476746136 0.00133799988507366 0.00286900545038753]  Capacitance=[8.11484299003193e-09 -1.94249816214699e-09 -1.86930692621136e-09;-1.94249816214699e-09 8.0425699231653e-09 -1.98049571960044e-09;-1.86930692621136e-09 -1.98049571960044e-09 8.13337738722527e-09]  x1=[204.872907593175 6115.37930863852 6116.23759521471;314.159265358979 314.159265358979 314.159265358979;0.860066677010055 -0.316890115378831 -1.88834095708038]  x2=[204.872988148159 6115.36064023953 6116.21894302594;314.159265358979 314.159265358979 314.159265358979;0.860066035791518 -0.316892720619597 -1.88834354498718]  x3=[0.178798885790713 14.9579495993111 15.0795962590828;314.159265358979 314.159265358979 314.159265358979;0.853975117559917 -0.312382815702647 -1.88388364155326]  x4=[0.180577017822415 16.1830272998931 16.3051010575522;314.159265358979 314.159265358979 314.159265358979;0.866006784435128 -0.321129837872762 -1.8925369729508]  x5=2.90549191369399e-07  V1=[157.3 5077 5080;314.2 314.2 314.2;0.3107 -0.9147 -2.485]  V2=[157.3 5077 5080;314.2 314.2 314.2;0.3107 -0.9147 -2.485]  I1=[0.1365 11.99 12.09;314.2 314.2 314.2;0.3061 -0.889 -2.46]  I2=[0.1394 13.87 13.98;314.2 314.2 314.2;0.3151 -0.9369 -2.507]  nHarmo=1  Measurements=None  Decoupling=off  VsMag0=0  VrMag0=0  VsAngle0=0  VrAngle0=0  IsMag0=0  IrMag0=0  IsAngle0=0  IrAngle0=0
      settings: SourceProductBaseCode=PS
  Line 7 : spsDistributedParametersLineLib/Distributed Parameters Line  Phases=3  Length=0.13  Frequency=50  Resistance=[0.476003738225748 0.351747138225748 0.351747138225748;0.351747138225748 0.476003738225748 0.351747138225748;0.351747138225748 0.351747138225748 0.476003738225748]  Inductance=[0.000705954362986426 0.000459934243504405 0.000459934243504405;0.000459934243504405 0.000705954362986426 0.000459934243504405;0.000459934243504405 0.000459934243504405 0.000705954362986426]  Capacitance=[5.7561313269996e-07 -1.37543883484145e-07 -1.37543912800485e-07;-1.37543883484145e-07 5.75613027339387e-07 -1.37543875208088e-07;-1.37543912800485e-07 -1.37543875208088e-07 5.75613005057695e-07]  x1=[60.7299447558302 6116.24787508195 6117.37256594239;314.159265358979 314.159265358979 314.159265358979;0.867537462170605 -0.24192885315373 -1.81323361981337]  x2=[60.7299695019387 6116.23639770868 6117.36108645846;314.159265358979 314.159265358979 314.159265358979;0.867536521225275 -0.241929443440024 -1.81323421009962]  x3=[0.824381015402819 328.473468119715 328.533844283292;314.159265358979 314.159265358979 314.159265358979;0.866634254791871 -0.241720579865101 -1.81302534642323]  x4=[0.824381006782856 329.697504114414 329.758105360726;314.159265358979 314.159265358979 314.159265358979;0.867536502157197 -0.242677023021752 -1.81398178974032]  x5=2.87356129084973e-06  V1=[38.27 5077 5081;314.2 314.2 314.2;0.4695 -0.8397 -2.41]  V2=[38.27 5077 5081;314.2 314.2 314.2;0.4695 -0.8397 -2.41]  I1=[0.5195 272.2 272.5;314.2 314.2 314.2;0.4686 -0.8385 -2.409]  I2=[0.5195 274.1 274.3;314.2 314.2 314.2;0.4695 -0.8413 -2.412]  nHarmo=1  Measurements=None  Decoupling=off  VsMag0=0  VrMag0=0  VsAngle0=0  VrAngle0=0  IsMag0=0  IrMag0=0  IsAngle0=0  IrAngle0=0
      settings: SourceProductBaseCode=PS
  Line 8 : spsDistributedParametersLineLib/Distributed Parameters Line  Phases=3  Length=1.19  Frequency=50  Resistance=[0.502970710632245 0.0486237908083191 0.0486712220507153;0.0486237908083191 0.502875844822084 0.0486237934466192;0.0486712220507153 0.0486237934466192 0.502970710632245]  Inductance=[0.00286900545038753 0.00133270803418135 0.00132951476746136;0.00133270803418135 0.00286931445999602 0.00133799988507366;0.00132951476746136 0.00133799988507366 0.00286900545038753]  Capacitance=[8.11484299003193e-09 -1.94249816214699e-09 -1.86930692621136e-09;-1.94249816214699e-09 8.0425699231653e-09 -1.98049571960044e-09;-1.86930692621136e-09 -1.98049571960044e-09 8.13337738722527e-09]  x1=[204.872544447172 6115.88361830447 6116.74102091159;314.159265358979 314.159265358979 314.159265358979;0.858360777737845 -0.318237069052544 -1.88968985579348]  x2=[202.750210342539 5073.03837892235 5074.76675240275;314.159265358979 314.159265358979 314.159265358979;0.838665313478345 -0.353946778634106 -1.92534727278734]  x3=[1.90172130585237 1330.95590031399 1334.46610015824;314.159265358979 314.159265358979 314.159265358979;-2.46232135729317 2.17074614610766 0.602396636124791]  x4=[2.25479374601164 1353.95862472976 1357.7028304278;314.159265358979 314.159265358979 314.159265358979;0.705833924313218 -0.958367966623379 -2.52670589416403]  x5=5.76255896215976e-06  V1=[157.3 5078 5081;314.2 314.2 314.2;0.309 -0.916 -2.486]  V2=[157.3 5068 5071;314.2 314.2 314.2;0.3086 -0.9171 -2.487]  I1=[0.1138 4.051 4.043;314.2 314.2 314.2;0.2108 0.8236 -0.7699]  I2=[0.1629 26.79 26.91;314.2 314.2 314.2;0.3758 -1.067 -2.637]  nHarmo=1  Measurements=None  Decoupling=off  VsMag0=0  VrMag0=0  VsAngle0=0  VrAngle0=0  IsMag0=0  IrMag0=0  IsAngle0=0  IrAngle0=0
      settings: SourceProductBaseCode=PS
  Line 9 : spsDistributedParametersLineLib/Distributed Parameters Line  Phases=3  Length=0.01  Frequency=50  Resistance=[0.646656091154803 0.0486237908083191 0.0486712220507153;0.0486237908083191 0.646561225344642 0.0486237934466192;0.0486712220507153 0.0486237934466192 0.646656091154803]  Inductance=[0.00282448912315926 0.00133270803418135 0.00132951476746136;0.00133270803418135 0.00282479813276775 0.00133799988507366;0.00132951476746136 0.00133799988507366 0.00282448912315926]  Capacitance=[7.89543174552926e-09 -1.85986777702161e-09 -1.7901190036642e-09;-1.85986777702161e-09 7.82540023894543e-09 -1.8957321828871e-09;-1.7901190036642e-09 -1.8957321828871e-09 7.91264394645417e-09]  x1=[149.213225790778 5073.09179697526 5075.1684030107;314.159265358979 314.159265358979 314.159265358979;0.854607401386096 -0.358699795443853 -1.93011429989817]  x2=[149.213231818881 5073.0909082083 5075.16751554225;314.159265358979 314.159265358979 314.159265358979;0.854607419017715 -0.358699833660442 -1.93011433752394]  x3=[0.13071809390334 12.8027747882706 12.9071768475146;314.159265358979 314.159265358979 314.159265358979;0.852766440754052 -0.354630263147953 -1.92607813784921]  x4=[0.130205761640112 13.0180626360481 13.1226242551289;314.159265358979 314.159265358979 314.159265358979;0.85644054074796 -0.362713924539617 -1.93409610482966]  x5=4.79147271261115e-08  V1=[104 5068 5071;314.2 314.2 314.2;0.3472 -0.9219 -2.492]  V2=[104 5068 5071;314.2 314.2 314.2;0.3472 -0.9219 -2.492]  I1=[0.09157 12.6 12.71;314.2 314.2 314.2;0.3397 -0.9106 -2.481]  I2=[0.09025 13.19 13.3;314.2 314.2 314.2;0.3549 -0.9326 -2.503]  nHarmo=1  Measurements=None  Decoupling=off  VsMag0=0  VrMag0=0  VsAngle0=0  VrAngle0=0  IsMag0=0  IrMag0=0  IsAngle0=0  IrAngle0=0
      settings: SourceProductBaseCode=PS
  Line im1 : spsDistributedParametersLineLib/Distributed Parameters Line  Phases=3  Length=1e-10  Frequency=50  Resistance=[0.646656091154803 0.0486237908083191 0.0486712220507153;0.0486237908083191 0.646561225344642 0.0486237934466192;0.0486712220507153 0.0486237934466192 0.646656091154803]  Inductance=[0.00282448912315926 0.00133270803418135 0.00132951476746136;0.00133270803418135 0.00282479813276775 0.00133799988507366;0.00132951476746136 0.00133799988507366 0.00282448912315926]  Capacitance=[7.89543174552926e-09 -1.85986777702161e-09 -1.7901190036642e-09;-1.85986777702161e-09 7.82540023894543e-09 -1.8957321828871e-09;-1.7901190036642e-09 -1.8957321828871e-09 7.91264394645417e-09]  x1=[182.880070226775 1341.37624017122 1345.22434166037;314.159265358979 314.159265358979 314.159265358979;0.816110193953804 -0.968336308131834 -2.53713356821093]  x2=[182.880070226776 1341.37624017114 1345.22434166028;314.159265358979 314.159265358979 314.159265358979;0.816110193953806 -0.968336308131853 -2.53713356821095]  x3=[0.162591682585272 2.38843809167569 2.40714846586195;314.159265358979 314.159265358979 314.159265358979;0.791490372246812 -0.796946076193134 -2.36054015512563]  x4=[0.157246436198661 4.49290594382928 4.54960993666129;314.159265358979 314.159265358979 314.159265358979;0.836131722472605 -1.0596598495874 -2.63042545113467]  x5=4.79147271261115e-16  V1=[104.3 5036 5039;314.2 314.2 314.2;0.3471 -0.9256 -2.496]  V2=[104.3 5036 5039;314.2 314.2 314.2;0.3471 -0.9256 -2.496]  I1=[0.1149 7.004 7.142;314.2 314.2 314.2;0.4879 -0.4472 -2.04]  I2=[0.06723 19.68 19.68;314.2 314.2 314.2;0.07907 -1.09 -2.656]  nHarmo=1  Measurements=None  Decoupling=off  VsMag0=0  VrMag0=0  VsAngle0=0  VrAngle0=0  IsMag0=0  IrMag0=0  IsAngle0=0  IrAngle0=0
      settings: SourceProductBaseCode=PS
  Load 174 : spsThreePhaseSeriesRLCLoadLib/Three-Phase Series RLC Load  LConnTagsString=A|B|C  Configuration=Delta  NominalVoltage=10000  Vabc=[1e3 1e3 1e3]  Vabcp=[1e3 1e3 1e3]  NominalFrequency=50  UnbalancedPower=off  ActivePower=6644.0013  InductivePower=4375.2483  CapacitivePower=0  Pabc=[10e3 9e3 11e3]  QLabc=[100 90 110]  QCabc=[100 90 110]  Pabcp=[10e3 9e3 11e3]  QLabcp=[100 90 110]  QCabcp=[100 90 110]  Measurements=None  LoadType=constant Z
  Load 178 : spsThreePhaseSeriesRLCLoadLib/Three-Phase Series RLC Load  LConnTagsString=A|B|C  Configuration=Delta  NominalVoltage=10000  Vabc=[1e3 1e3 1e3]  Vabcp=[1e3 1e3 1e3]  NominalFrequency=50  UnbalancedPower=off  ActivePower=2397.2302  InductivePower=1196.8054  CapacitivePower=0  Pabc=[10e3 9e3 11e3]  QLabc=[100 90 110]  QCabc=[100 90 110]  Pabcp=[10e3 9e3 11e3]  QLabcp=[100 90 110]  QCabcp=[100 90 110]  Measurements=None  LoadType=constant Z
  Load 1873 : spsThreePhaseSeriesRLCLoadLib/Three-Phase Series RLC Load  LConnTagsString=A|B|C  Configuration=Delta  NominalVoltage=10000  Vabc=[1e3 1e3 1e3]  Vabcp=[1e3 1e3 1e3]  NominalFrequency=50  UnbalancedPower=off  ActivePower=2293.6414  InductivePower=1310.764  CapacitivePower=0  Pabc=[10e3 9e3 11e3]  QLabc=[100 90 110]  QCabc=[100 90 110]  Pabcp=[10e3 9e3 11e3]  QLabcp=[100 90 110]  QCabcp=[100 90 110]  Measurements=None  LoadType=constant Z
  Load 534 : spsThreePhaseSeriesRLCLoadLib/Three-Phase Series RLC Load  LConnTagsString=A|B|C  Configuration=Delta  NominalVoltage=10000  Vabc=[1e3 1e3 1e3]  Vabcp=[1e3 1e3 1e3]  NominalFrequency=50  UnbalancedPower=off  ActivePower=17310.4266  InductivePower=11256.0499  CapacitivePower=0  Pabc=[10e3 9e3 11e3]  QLabc=[100 90 110]  QCabc=[100 90 110]  Pabcp=[10e3 9e3 11e3]  QLabcp=[100 90 110]  QCabcp=[100 90 110]  Measurements=None  LoadType=constant Z
  Load 535 : spsThreePhaseSeriesRLCLoadLib/Three-Phase Series RLC Load  LConnTagsString=A|B|C  Configuration=Delta  NominalVoltage=10000  Vabc=[1e3 1e3 1e3]  Vabcp=[1e3 1e3 1e3]  NominalFrequency=50  UnbalancedPower=off  ActivePower=9735.7818  InductivePower=6070.259  CapacitivePower=0  Pabc=[10e3 9e3 11e3]  QLabc=[100 90 110]  QCabc=[100 90 110]  Pabcp=[10e3 9e3 11e3]  QLabcp=[100 90 110]  QCabcp=[100 90 110]  Measurements=None  LoadType=constant Z
  Load 8042 : spsThreePhaseSeriesRLCLoadLib/Three-Phase Series RLC Load  LConnTagsString=A|B|C  Configuration=Delta  NominalVoltage=10000  Vabc=[1e3 1e3 1e3]  Vabcp=[1e3 1e3 1e3]  NominalFrequency=50  UnbalancedPower=off  ActivePower=1006.297  InductivePower=613.553  CapacitivePower=0  Pabc=[10e3 9e3 11e3]  QLabc=[100 90 110]  QCabc=[100 90 110]  Pabcp=[10e3 9e3 11e3]  QLabcp=[100 90 110]  QCabcp=[100 90 110]  Measurements=None  LoadType=constant Z
  Load 8131 : spsThreePhaseSeriesRLCLoadLib/Three-Phase Series RLC Load  LConnTagsString=A|B|C  Configuration=Delta  NominalVoltage=10000  Vabc=[1e3 1e3 1e3]  Vabcp=[1e3 1e3 1e3]  NominalFrequency=50  UnbalancedPower=off  ActivePower=26372.175  InductivePower=18529.6749  CapacitivePower=0  Pabc=[10e3 9e3 11e3]  QLabc=[100 90 110]  QCabc=[100 90 110]  Pabcp=[10e3 9e3 11e3]  QLabcp=[100 90 110]  QCabcp=[100 90 110]  Measurements=None  LoadType=constant Z
  Load 8429 : spsThreePhaseSeriesRLCLoadLib/Three-Phase Series RLC Load  LConnTagsString=A|B|C  Configuration=Delta  NominalVoltage=10000  Vabc=[1e3 1e3 1e3]  Vabcp=[1e3 1e3 1e3]  NominalFrequency=50  UnbalancedPower=off  ActivePower=6691.7956  InductivePower=2704.2118  CapacitivePower=0  Pabc=[10e3 9e3 11e3]  QLabc=[100 90 110]  QCabc=[100 90 110]  Pabcp=[10e3 9e3 11e3]  QLabcp=[100 90 110]  QCabcp=[100 90 110]  Measurements=None  LoadType=constant Z
  Load 894 : spsThreePhaseSeriesRLCLoadLib/Three-Phase Series RLC Load  LConnTagsString=A|B|C  Configuration=Delta  NominalVoltage=10000  Vabc=[1e3 1e3 1e3]  Vabcp=[1e3 1e3 1e3]  NominalFrequency=50  UnbalancedPower=off  ActivePower=3246.7774  InductivePower=1258.5349  CapacitivePower=0  Pabc=[10e3 9e3 11e3]  QLabc=[100 90 110]  QCabc=[100 90 110]  Pabcp=[10e3 9e3 11e3]  QLabcp=[100 90 110]  QCabcp=[100 90 110]  Measurements=None  LoadType=constant Z
  Load 895 : spsThreePhaseSeriesRLCLoadLib/Three-Phase Series RLC Load  LConnTagsString=A|B|C  Configuration=Delta  NominalVoltage=10000  Vabc=[1e3 1e3 1e3]  Vabcp=[1e3 1e3 1e3]  NominalFrequency=50  UnbalancedPower=off  ActivePower=1257.9477  InductivePower=324.0486  CapacitivePower=0  Pabc=[10e3 9e3 11e3]  QLabc=[100 90 110]  QCabc=[100 90 110]  Pabcp=[10e3 9e3 11e3]  QLabcp=[100 90 110]  QCabcp=[100 90 110]  Measurements=None  LoadType=constant Z
  R1 : spsThreePhaseVIMeasurementLib/Three-Phase V-I Measurement  VoltageMeasurement=phase-to-ground  SetLabelV=off  LabelV=Vabc  Vpu=off  VpuLL=off  CurrentMeasurement=yes  SetLabelI=off  LabelI=Iabc  Ipu=off  Pbase=100e6  Vbase=500e3  OutputType=Complex  PhasorSimulation=on  PSBequivalent=0
  R4 : spsThreePhaseVIMeasurementLib/Three-Phase V-I Measurement  VoltageMeasurement=phase-to-ground  SetLabelV=off  LabelV=Vabc  Vpu=off  VpuLL=off  CurrentMeasurement=yes  SetLabelI=off  LabelI=Iabc  Ipu=off  Pbase=100e6  Vbase=500e3  OutputType=Complex  PhasorSimulation=on  PSBequivalent=0
  Scope R1 : Scope  NumInputPorts=2
  Scope R4 : Scope  NumInputPorts=2
  Source PC1_TT2 : spsThreePhaseSourceLib/Three-Phase Source  InternalConnection=Yn  VoltagePhases=off  Voltage=10000  PhaseAngle=0  Voltage_phases=[25e3 25e3 25e3]/sqrt(3)  PhaseAngles_phases=[0 -120 +120]  Frequency=50  NonIdealSource=on  SpecifyImpedance=off  Resistance=0.14  Inductance=0.0031831  ShortCircuitLevel=100e6  BaseVoltage=25e3  XRratio=7  BusType=swing  Pref=10e3  Qref=0  Prefabc=[10e3, 10e3, 10e3]  Qrefabc=[0, 0, 0]  Qmin=-inf  Qmax=inf
  Source Zn : spsSeriesRLCBranchLib/Series RLC Branch  LConnTagsString=__new0  RConnTagsString=__new0  BranchType=RL  Resistance=0.001  Inductance=3.1831e-06  SetiL0=off  InitialCurrent=0  Capacitance=0  Setx0=off  InitialVoltage=0  Measurements=None
  powergui : spspowerguiLib/powergui  Priority=1  SimulationMode=Phasor  SampleTime=50e-6  frequency=50  Iterations=50  frequencyindice=50  Pbase=100e6  ErrMax=1e-4  UnitsV=kV  UnitsW=MW  buscounter=0  FunctionMessages=off  echomessages=off  EnableUseOfTLC=off  CurrentSourceSwitches=off  DisableSnubberDevices=off  DisableRonSwitches=off  DisableVfSwitches=off  DisplayEquations=off  AutomaticDiscreteSolvers=off  SolverType=Tustin/Backward Euler (TBE)  Interpol=off  ExternalGateDelay=off  methode=off  Ts=10  x0status=blocks  SPID=off  SwTol=0  HookPort=off  NonlinearTolerance=1e-4  nMaxIteration=100  ContinueOnMaxIteration=off  RestoreLinks=warning  ResistiveCurrentMeasurement=off  Frange=[0:2:500]  Ylog=off  Xlog=on  ShowGrid=off  save=off  variable=ZData  structure=0  ZoomFFT=off  StartTime=0.0  cycles=1  DisplayStyle=1  fundamental=60  FreqAxis=off  MaxFrequency=1000  frequencyindicesteady=1  RmsSteady=1  display=off
  wires:
  R1/2 -> Scope R1/2
  R1/1 -> Scope R1/1
  R4/1 -> Scope R4/1
  R4/2 -> Scope R4/2
  connections:
  Line 15/RConn2 -- Line 17/LConn2 -- Line 16/LConn2
  Line 8/RConn3 -- Line 15/LConn3 -- Line 10/LConn3 -- Line 9/LConn3
  Line 4/RConn1 -- Line 6/LConn1 -- Line 5/LConn1
  Line 3/RConn2 -- Line 8/LConn2 -- Line 4/LConn2
  Line 3/RConn3 -- Line 8/LConn3 -- Line 4/LConn3
  Line 10/RConn2 -- Line 11/LConn2 -- Line 12/LConn2
  Line 17/RConn1 -- Line 34/LConn1 -- Line 18/LConn1
  Line im1/RConn3 -- Line 35/LConn3 -- Load 8131/LConn3
  Line 12/RConn3 -- Line 14/LConn3 -- Line 13/LConn3
  Line 2/RConn2 -- Load 178/LConn2 -- Line 3/LConn2
  Line 2/RConn3 -- Load 178/LConn3 -- Line 3/LConn3
  Line 15/RConn3 -- Line 17/LConn3 -- Line 16/LConn3
  Line 19/RConn1 -- Load 8429/LConn1
  Line 10/RConn1 -- Line 11/LConn1 -- Line 12/LConn1
  Line 8/RConn2 -- Line 15/LConn2 -- Line 10/LConn2 -- Line 9/LConn2
  Line 8/RConn1 -- Line 15/LConn1 -- Line 10/LConn1 -- Line 9/LConn1
  Line 4/RConn3 -- Line 6/LConn3 -- Line 5/LConn3
  Line 3/RConn1 -- Line 8/LConn1 -- Line 4/LConn1
  Line 10/RConn3 -- Line 11/LConn3 -- Line 12/LConn3
  Line 4/RConn2 -- Line 6/LConn2 -- Line 5/LConn2
  Line 17/RConn2 -- Line 34/LConn2 -- Line 18/LConn2
  Line 17/RConn3 -- Line 34/LConn3 -- Line 18/LConn3
  Line 19/RConn3 -- Load 8429/LConn3
  Line 19/RConn2 -- Load 8429/LConn2
  Line im1/RConn2 -- Line 35/LConn2 -- Load 8131/LConn2
  Line 2/RConn1 -- Load 178/LConn1 -- Line 3/LConn1
  Line 15/RConn1 -- Line 17/LConn1 -- Line 16/LConn1
  Line 12/RConn1 -- Line 14/LConn1 -- Line 13/LConn1
  Line im1/RConn1 -- Line 35/LConn1 -- Load 8131/LConn1
  Line 12/RConn2 -- Line 14/LConn2 -- Line 13/LConn2
  Line 34/RConn3 -- R4/LConn3
  Load 1873/LConn2 -- Line 9/RConn2
  Line 11/RConn1 -- Load 174/LConn1
  Line 36/LConn3 -- Line 35/RConn3
  Line 7/RConn3 -- Load 535/LConn3
  Line 34/RConn2 -- R4/LConn2
  Line 34/RConn1 -- R4/LConn1
  Line 7/RConn1 -- Load 535/LConn1
  Line 36/LConn1 -- Line 35/RConn1
  Line 18/RConn1 -- Line 19/LConn1
  Line im1/LConn1 -- R4/RConn1
  Line 36/LConn2 -- Line 35/RConn2
  Line 7/LConn1 -- Line 6/RConn1
  Line 18/RConn2 -- Line 19/LConn2
  Line 7/LConn2 -- Line 6/RConn2
  Line 5/RConn2 -- Load 534/LConn2
  Source PC1_TT2/RConn1 -- Line/LConn1
  Load 8042/LConn3 -- Line 16/RConn3
  Line 14/RConn2 -- Load 895/LConn2
  Load 1873/LConn3 -- Line 9/RConn3
  Load 8042/LConn2 -- Line 16/RConn2
  Load 1873/LConn1 -- Line 9/RConn1
  Line im1/LConn2 -- R4/RConn2
  Line 5/RConn3 -- Load 534/LConn3
  Line/RConn1 -- R1/LConn1
  Line 2/LConn3 -- R1/RConn3
  Line 13/RConn3 -- Load 894/LConn3
  Source Zn/RConn1 -- Source PC1_TT2/LConn1
  Line 11/RConn2 -- Load 174/LConn2
  Line 14/RConn1 -- Load 895/LConn1
  Source PC1_TT2/RConn2 -- Line/LConn2
  Line/RConn3 -- R1/LConn3
  Ground/LConn1 -- Source Zn/LConn1
  Line 18/RConn3 -- Line 19/LConn3
  Load 8042/LConn1 -- Line 16/RConn1
  Line 11/RConn3 -- Load 174/LConn3
  Line 2/LConn1 -- R1/RConn1
  Line 14/RConn3 -- Load 895/LConn3
  Line 2/LConn2 -- R1/RConn2
  Line 5/RConn1 -- Load 534/LConn1
  Line im1/LConn3 -- R4/RConn3
  Line/RConn2 -- R1/LConn2
  Line 7/LConn3 -- Line 6/RConn3
  Line 13/RConn2 -- Load 894/LConn2
  Line 13/RConn1 -- Load 894/LConn1
  Source PC1_TT2/RConn3 -- Line/LConn3
  Line 7/RConn2 -- Load 535/LConn2
